simulink model "Problema2"  (R2023b)
settings: Solver=VariableStepAuto  StartTime=0.0  StopTime=30  RelTol=1e-3
undefined symbols (not defined in the file): m
settings Model: Creator=alfre  LastModifiedBy=alfre

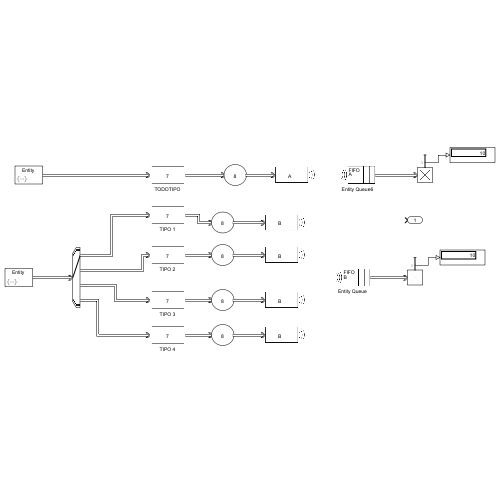
[thumbnail: Simulink's stored preview of the top-level diagram]
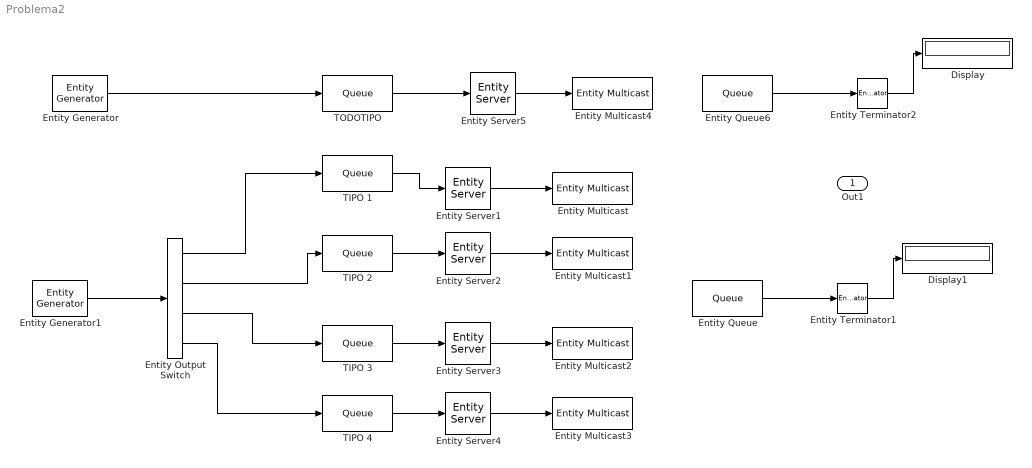
== system Problema2 ==
  Display : Display
  Display1 : Display
  Entity Output Switch : EntityOutputSwitch  InputPortMessageModes=m  OutputPortMessageModes=m,m,m,m  NumberOutputPorts=4  SwitchAttributeName=Attribute1
      settings: OutputPortMap=o0,o1,o2,o3
  Entity Generator : EntityGenerator  OutputPortMessageModes=m  TimeSource=MATLAB action  IntergenerationTimeAction=|  GenerateAction=|  AttributeName=Type|ServiceTime  AttributeInitialValue=0|0  EntityType=Structured  EntityTypeName=Entity
      IntergenerationTimeAction=|
      | persistent rngInit;
      | if isempty(rngInit)
      |     seed = 12345;
      |     rng(seed);
      |     rngInit = true;
      | end
      | 
      | % Pattern: Poisson distribution
      | % m: Mean
      | m = 2;
      | dt = poissrnd(m);
      GenerateAction=|
      | % 4 tipos de barcos (1, 2, 3 y 4)
      | entity.Type = randi([1, 4], 1, 1)
      | % El tiempo de reparación de un barco i
      | % Se obtiene de una distribución de poisson
      | % de lambda = i = tipo
      | entity.ServiceTime = poissrnd(entity.Type)
  Entity Generator1 : EntityGenerator  OutputPortMessageModes=m  TimeSource=MATLAB action  IntergenerationTimeAction=|  GenerateAction=|  AttributeName=Type|ServiceTime  AttributeInitialValue=0|0  EntityType=Structured  EntityTypeName=Entity
      IntergenerationTimeAction=|
      | persistent rngInit;
      | if isempty(rngInit)
      |     seed = 12345;
      |     rng(seed);
      |     rngInit = true;
      | end
      | 
      | % Pattern: Poisson distribution
      | % m: Mean
      | m = 2;
      | dt = poissrnd(m);
      GenerateAction=|
      | % 4 tipos de barcos (1, 2, 3 y 4)
      | entity.Type = randi([1, 4], 1, 1)
      | % El tiempo de reparación de un barco i
      | % Se obtiene de una distribución de poisson
      | % de lambda = i = tipo
      | entity.ServiceTime = poissrnd(entity.Type)
  Entity Multicast{,1..3} (4 alike) : EntityMulticast  Tag=B  InputPortMessageModes=m  MulticastTag=B
  Entity Multicast4 : EntityMulticast  Tag=A  InputPortMessageModes=m
  Entity Queue : Queue  OutputPortMessageModes=m  EntityArrivalSource=Multicast  MulticastTag=B
  Entity Queue6 : Queue  OutputPortMessageModes=m  EntityArrivalSource=Multicast
  Entity Server{1..5} (5 alike) : EntityServer  InputPortMessageModes=m  OutputPortMessageModes=m  Capacity=8  ServiceTimeSource=Attribute  ServiceTimeAction=if entity
  Entity Terminator1 : EntityTerminator  InputPortMessageModes=m  NumberEntitiesArrived=on
      settings: OutputPortMap=o0
  Entity Terminator2 : EntityTerminator  InputPortMessageModes=m  NumberEntitiesArrived=on
      settings: OutputPortMap=o0
  TIPO 1 : Queue  InputPortMessageModes=m  OutputPortMessageModes=m  OverwriteOldest=on  Capacity=7  AverageQueueLength=on
  TIPO 2 : Queue  InputPortMessageModes=m  OutputPortMessageModes=m  OverwriteOldest=on  Capacity=7
  TIPO 3 : Queue  InputPortMessageModes=m  OutputPortMessageModes=m  OverwriteOldest=on  Capacity=7
  TIPO 4 : Queue  InputPortMessageModes=m  OutputPortMessageModes=m  OverwriteOldest=on  Capacity=7
  TODOTIPO : Queue  InputPortMessageModes=m  OutputPortMessageModes=m  OverwriteOldest=on  Capacity=7
  Out1 : Outport
  wires:
  Entity Generator/1 -> TODOTIPO/1
  Entity Output Switch/1 -> TIPO 1/1
  Entity Output Switch/2 -> TIPO 2/1
  Entity Output Switch/3 -> TIPO 3/1
  Entity Output Switch/4 -> TIPO 4/1
  Entity Generator1/1 -> Entity Output Switch/1
  Entity Server1/1 -> Entity Multicast/1
  Entity Server4/1 -> Entity Multicast3/1
  Entity Server3/1 -> Entity Multicast2/1
  Entity Server2/1 -> Entity Multicast1/1
  Entity Queue/1 -> Entity Terminator1/1
  TIPO 1/1 -> Entity Server1/1
  TIPO 2/1 -> Entity Server2/1
  TIPO 3/1 -> Entity Server3/1
  TIPO 4/1 -> Entity Server4/1
  TODOTIPO/1 -> Entity Server5/1
  Entity Server5/1 -> Entity Multicast4/1
  Entity Queue6/1 -> Entity Terminator2/1
  Entity Terminator2/1 -> Display/1
  Entity Terminator1/1 -> Display1/1
